simulink model "forward"  (R2016b)
settings: Solver=ode3  StartTime=0.0  StopTime=mdl.tEnd  FixedStep=mdl.tStep  RelTol=1e-3
undefined symbols (not defined in the file): magnitude, pto, ss
settings Model: Creator=ggparker  LastModifiedBy=s1343354
settings DataIOCC: SaveFinalState=on  SaveCompleteFinalSimState=on  SaveOutput=off  SaveTime=off

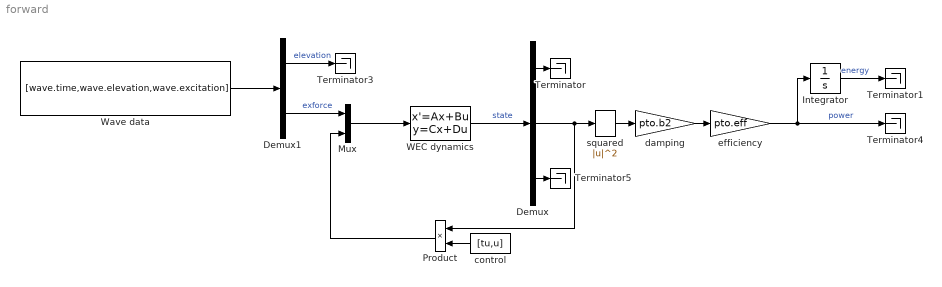
== system forward ==
  Demux : Demux  Outputs=[3; 1; 4]
  Demux1 : Demux  Outputs=[1; 1]
  Integrator : Integrator
  Mux : Mux  Inputs=2
  Product : Product
  Terminator{,1,3..5} (5 alike) : Terminator
  WEC dynamics : StateSpace  A=ss.A  B=ss.B  C=ss.C  D=ss.D  X0=0
  Wave data : FromWorkspace  VariableName=[wave.time,wave.elevation,wave.excitation]  SampleTime=0
  control : FromWorkspace  VariableName=[tu,u]  SampleTime=0  Interpolate=off  OutputAfterFinalValue=Holding final value
  damping : Gain  Gain=pto.b2
  efficiency : Gain  Gain=pto.eff
  squared : Math  Operator=magnitude^2  SaturateOnIntegerOverflow=on
  wires:
  efficiency/1 -> Terminator4/1, Integrator/1  "power"
  WEC dynamics/1 -> Demux/1  "state"
  Wave data/1 -> Demux1/1
  Demux1/1 -> Terminator3/1  "elevation"
  Integrator/1 -> Terminator1/1  "energy"
  Demux1/2 -> Mux/1  "exforce"
  damping/1 -> efficiency/1
  Demux/2 -> Product/1, squared/1
  Demux/1 -> Terminator/1
  Demux/3 -> Terminator5/1
  squared/1 -> damping/1
  Mux/1 -> WEC dynamics/1
  control/1 -> Product/2
  Product/1 -> Mux/2
